simulink model "motor_car"  (R2023b)
settings: Solver=ode1  StartTime=0.0  StopTime=20  FixedStep=0.001  RelTol=1e-3
values from neighbouring files (symbols this model uses):
  b = 3.97e-6    (= 3.97e-06)    [parameters.m]
  g = 9.81    [parameters.m]
  GR = 3.42    [parameters.m]
  i_0 = 0    [parameters.m]
  J = 0.0421    [parameters.m]
  Kb = 0.6970    (= 0.697)    [parameters.m]
  Km = Kb    (= 0.697)    [parameters.m]
  L = 177e-6    (= 0.000177)    [parameters.m]
  m = 250    [parameters.m]
  Q = 0.5    [parameters.m]
  R = 0.018    [parameters.m]
  Rw = 0.1778    [parameters.m]
  tht_0 = 0    [parameters.m]
  tol = 1.0e-10    (= 1e-10)    [parameters.m]
  v_0 = 0    [parameters.m]
  wm_0 = 0    [parameters.m]
  wm_des = 275    [parameters.m]
  xp_0 = 0    [parameters.m]
libraries: simulink x1
settings Model: Creator=nikkparasar  LastModifiedBy=nikkparasar

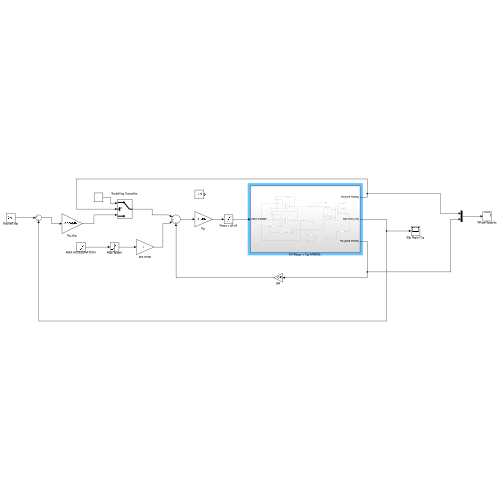
[thumbnail: Simulink's stored preview of the top-level diagram]
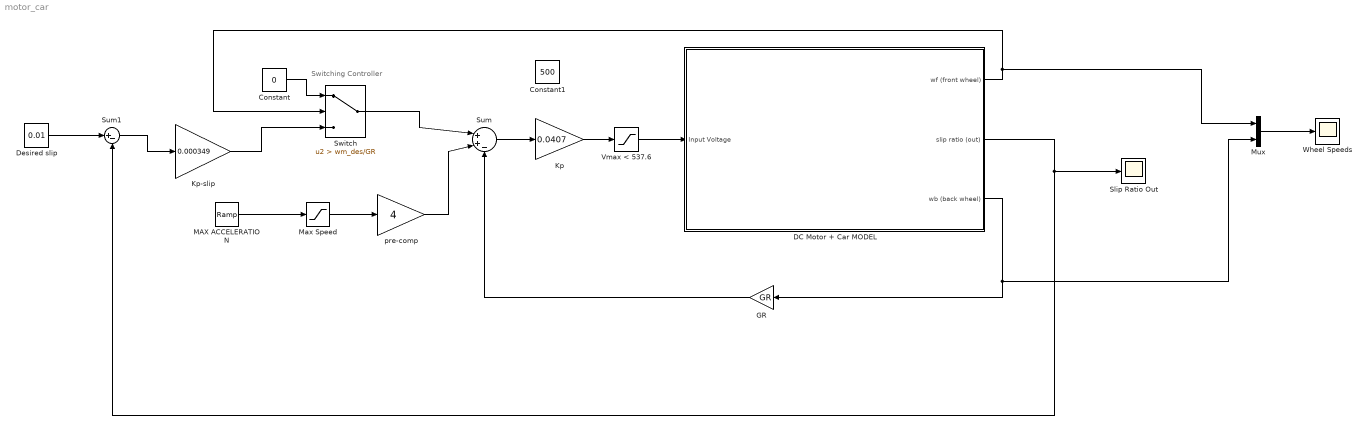
== system motor_car ==
  note: Switching Controller
  Constant : Constant  Value=0
  Constant1 : Constant  Value=500
  DC Motor + Car MODEL : Subsystem
  Desired slip : Constant  Value=0.01
  GR : Gain  Gain=GR
  Kp : Gain  Gain=0.0407
  Kp-slip : Gain  Gain=0.000349
  MAX ACCELERATION : simulink/Sources/Ramp  slope=50  start=0  InitialOutput=0
  Max Speed : Saturate  UpperLimit=wm_des  LowerLimit=0
  Mux : Mux  Inputs=2
  Slip Ratio Out : Scope
  Sum : Sum  Inputs=|++-
  Sum1 : Sum  Inputs=|+-
  Switch : Switch  Criteria=u2 > Threshold  Threshold=wm_des/GR  SaturateOnIntegerOverflow=off  InputSameDT=off
  Vmax < 537.6 : Saturate  UpperLimit=537.6  LowerLimit=0
  Wheel Speeds : Scope
  pre-comp : Gain  Gain=4
  wires:
  DC Motor + Car MODEL/3(wb (back wheel)) -> GR/1, Mux/2
  Kp/1 -> Vmax < 537.6/1
  GR/1 -> Sum/3
  Sum/1 -> Kp/1
  Max Speed/1 -> pre-comp/1
  MAX ACCELERATION/1 -> Max Speed/1
  pre-comp/1 -> Sum/2
  Switch/1 -> Sum/1
  DC Motor + Car MODEL/1(wf (front wheel)) -> Mux/1, Switch/2
  Constant/1 -> Switch/1
  Sum1/1 -> Kp-slip/1
  Desired slip/1 -> Sum1/1
  DC Motor + Car MODEL/2(slip ratio (out)) -> Sum1/2, Slip Ratio Out/1
  Kp-slip/1 -> Switch/3
  Mux/1 -> Wheel Speeds/1
  Vmax < 537.6/1 -> DC Motor + Car MODEL/1(Input Voltage)

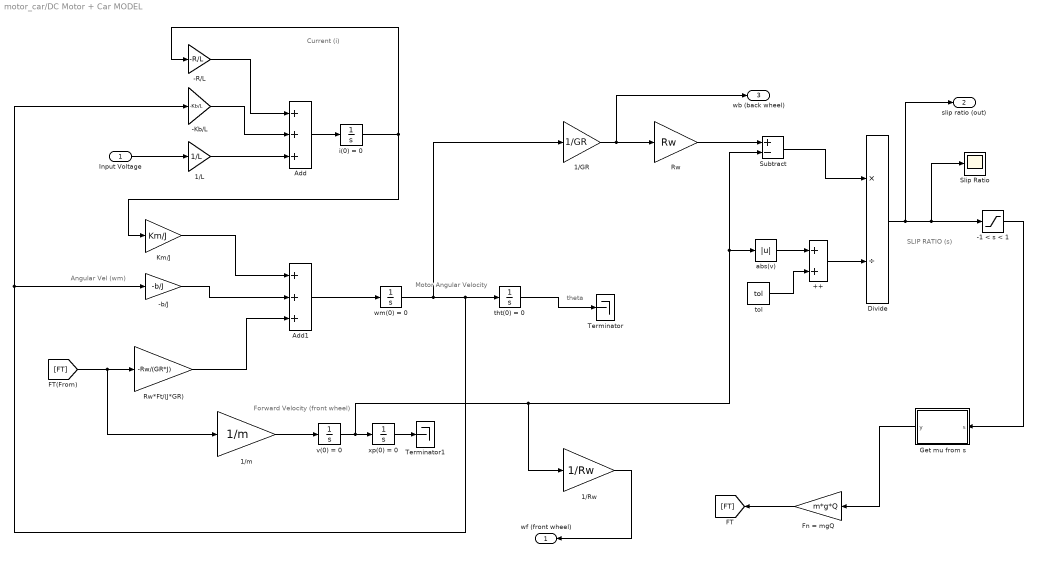
== system motor_car/DC Motor + Car MODEL ==
  note: SLIP RATIO (s)
  note: Forward Velocity (front wheel)
  note: theta
  note: Angular Vel (wm)
  note: Motor Angular Velocity
  note: Current (i)
  Input Voltage : Inport
  ++ : Sum
  -1 < s < 1 : Saturate  UpperLimit=1  LowerLimit=-1
  -Kb/L : Gain  Gain=-Kb/L
  -R/L : Gain  Gain=-R/L
  -b/J : Gain  Gain=-b/J
  1/GR : Gain  Gain=1/GR
  1/L : Gain  Gain=1/L
  1/Rw : Gain  Gain=1/Rw
  1/m : Gain  Gain=1/m
  Add : Sum  Inputs=+++
  Add1 : Sum  Inputs=+++
  Divide : Product  Inputs=*/  RndMeth=Zero  SaturateOnIntegerOverflow=on
  Fn = mgQ : Gain  Gain=m*g*Q
  Get mu from s : MATLAB Function  TreatAsAtomicUnit=on
  Km/J : Gain  Gain=Km/J
  Rw : Gain  Gain=Rw
  Rw*Ft/(J*GR) : Gain  Gain=-Rw/(GR*J)
  Slip Ratio : Scope
  Subtract : Sum  Inputs=+-
  Terminator : Terminator
  Terminator1 : Terminator
  abs(v) : Abs  SaturateOnIntegerOverflow=off
  i(0) = 0 : Integrator  InitialCondition=i_0
  tht(0) = 0 : Integrator  InitialCondition=tht_0
  tol : Constant  Value=tol
  v(0) = 0 : Integrator  InitialCondition=v_0
  wm(0) = 0 : Integrator  InitialCondition=wm_0
  "xp(0) = 0 " : Integrator  InitialCondition=xp_0
  wf (front wheel) : Outport
  slip ratio (out) : Outport  Port=2
  wb (back wheel) : Outport  Port=3
  wires:
  1/Rw/1 -> wf (front wheel)/1
  Divide/1 -> slip ratio (out)/1, Slip Ratio/1, -1 < s < 1/1
  Fn = mgQ/1 -> [FT]
  Add1/1 -> wm(0) = 0/1
  1/L/1 -> Add/3
  Rw*Ft/(J*GR)/1 -> Add1/3
  -Kb/L/1 -> Add/2
  tht(0) = 0/1 -> Terminator/1
  Add/1 -> i(0) = 0/1
  Input Voltage/1 -> 1/L/1
  -R/L/1 -> Add/1
  abs(v)/1 -> ++/1
  Get mu from s/1(y) -> Fn = mgQ/1
  1/m/1 -> v(0) = 0/1
  [FT] -> 1/m/1, Rw*Ft/(J*GR)/1
  ++/1 -> Divide/2
  Rw/1 -> Subtract/1
  i(0) = 0/1 -> -R/L/1, Km/J/1
  -1 < s < 1/1 -> Get mu from s/1(s)
  1/GR/1 -> wb (back wheel)/1, Rw/1
  -b/J/1 -> Add1/2
  Km/J/1 -> Add1/1
  wm(0) = 0/1 -> tht(0) = 0/1, -Kb/L/1, -b/J/1, 1/GR/1
  tol/1 -> ++/2
  v(0) = 0/1 -> 1/Rw/1, Subtract/2, abs(v)/1, "xp(0) = 0 "/1
  "xp(0) = 0 "/1 -> Terminator1/1
  Subtract/1 -> Divide/1

== matlab function motor_car/DC Motor + Car MODEL/Get mu from s ==
  data: s input; y output
function y = fcn(s)

% slip is already saturated
% ONLY DEFINED FROM 1 to -1

a1 = 1.63;
a2 = -0.9;
a3 = -0.1;

c1 = -27;
c2 = -15;

if s<0
    s = abs(s)
    mu = -(a1*(1-exp(c1*s))+a2*(1-exp(c2*s))+a3*s);
else
    mu = a1*(1-exp(c1*s))+a2*(1-exp(c2*s))+a3*s;
end

y = mu
